simulink model "Bdy"  (R2020b)
settings: configuration reference "unit_config" (kept outside this file)
undefined symbols (not defined in the file): Bdy_facTireFric_C, Bdy_lenRadiusWheel_C, Bdy_mEquivalentJ_C, Bdy_mVeh_C, Bdy_vsqr2frc_C
settings Model: DataDictionary=Hybrid_vehicle.sldd  SimulationMode=accelerator  Creator=Georg  LastModifiedBy=jy
settings ConfigSetRef: SourceName=unit_config

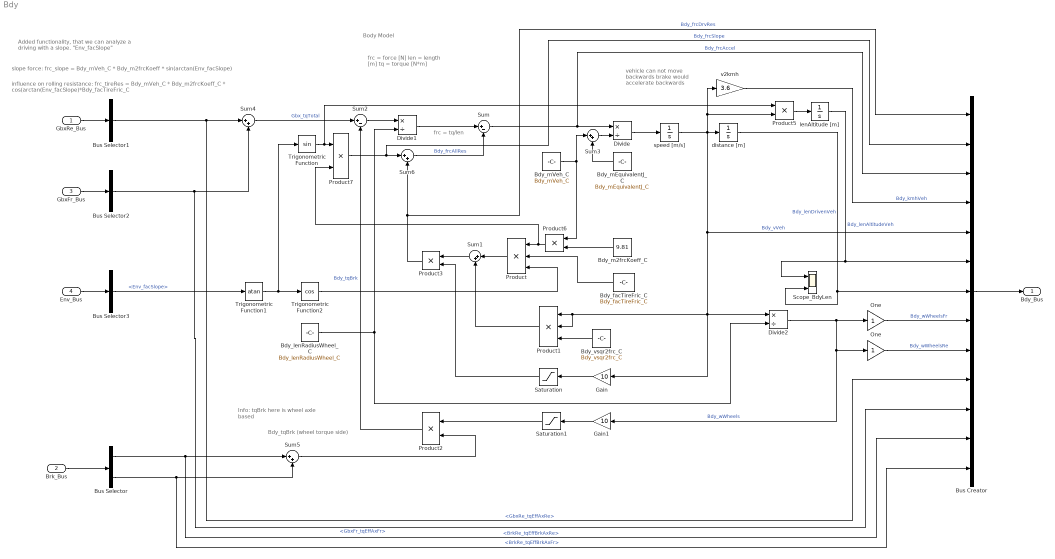
== system Bdy ==
  note: influence on rolling resistance: frc_tireRes = Bdy_mVeh_C * Bdy_m2frcKoeff_C * cos(arctan(Env_facSlope)*Bdy_facTireFric_C
  note: slope force: frc_slope = Bdy_mVeh_C * Bdy_m2frcKoeff * sin(arctan(Env_facSlope)
  note: Added functionality, that we can analyze a
      | driving with a slope.  "Env_facSlope"
  note: Info:
      | tqBrk here is wheel axle based
  note: Body Model
  note: Bdy_tqBrk
      | (wheel torque side)
  note: frc = tq/len
  note: vehicle can not
      | move backwards
      | brake would accelerate
      | backwards
  note: frc = force [N]
      | len = length [m]
      | tq = torque [N*m]
  GbxRe_Bus : Inport
  Brk_Bus : Inport  Port=2
  GbxFr_Bus : Inport  Port=3
  Env_Bus : Inport  Port=4
  Bdy_facTireFric_C : Constant  Value=Bdy_facTireFric_C
  Bdy_lenRadiusWheel_C : Constant  Value=Bdy_lenRadiusWheel_C
  Bdy_m2frcKoeff_C : Constant  Value=9.81
  Bdy_mEquivalentJ_C : Constant  Value=Bdy_mEquivalentJ_C
  Bdy_mVeh_C : Constant  Value=Bdy_mVeh_C
  Bdy_vsqr2frc_C : Constant  Value=Bdy_vsqr2frc_C
  Bus Creator : BusCreator  Inputs=13
  Bus Selector : BusSelector  OutputSignals=BrkRe_tqEffBrkAxRe,BrkRe_tqEffBrkAxFr
  Bus Selector1 : BusSelector  OutputSignals=GbxRe_tqEffAxRe
  Bus Selector2 : BusSelector  OutputSignals=GbxFr_tqEffAxFr
  Bus Selector3 : BusSelector  OutputSignals=Env_facSlope
  Divide : Product  Inputs=*/
  Divide1 : Product  Inputs=*/
  Divide2 : Product  Inputs=*/
  Gain : Gain  Gain=10
  Gain1 : Gain  Gain=10
  One : Gain
  "One " : Gain
  Product : Product  Inputs=3  RndMeth=Zero
  Product1 : Product  Inputs=3  RndMeth=Zero
  Product2 : Product  RndMeth=Zero
  Product3 : Product  RndMeth=Zero
  Product5 : Product
  Product6 : Product  RndMeth=Zero
  Product7 : Product
  Saturation : Saturate  UpperLimit=1  LowerLimit=-1
  Saturation1 : Saturate  UpperLimit=1  LowerLimit=-1
  "Scope_BdyLen  " : Scope  NumInputPorts=2
  Sum : Sum  Inputs=|+-
  Sum{1,3..6} (5 alike) : Sum  Inputs=|++
  Sum2 : Sum  Inputs=|+-
  Trigonometric Function : Trigonometry
  Trigonometric Function1 : Trigonometry  Operator=atan
  Trigonometric Function2 : Trigonometry  Operator=cos
  distance [m] : Integrator
  lenAltitude [m] : Integrator
  speed [m/s] : Integrator  LimitOutput=on  LowerSaturationLimit=0
  v2kmh : Gain  Gain=3.6
  Bdy_Bus : Outport  VectorParamsAs1DForOutWhenUnconnected=off
  wires:
  Divide/1 -> speed [m/s]/1
  Product6/1 -> Product7/2, Product/1
  lenAltitude [m]/1 -> "Scope_BdyLen  "/1, Bus Creator/6  "Bdy_lenAltitudeVeh"
  Product5/1 -> lenAltitude [m]/1
  Trigonometric Function2/1 -> Product/3
  One/1 -> Bus Creator/9  "Bdy_wWheelsRe"
  Bdy_lenRadiusWheel_C/1 -> Divide2/2, Divide1/2
  GbxFr_Bus/1 -> Bus Selector2/1
  Sum6/1 -> Sum/2  "Bdy_frcAllRes"
  Product/1 -> Sum1/1
  Trigonometric Function/1 -> Product5/1, Product7/1
  Bdy_mEquivalentJ_C/1 -> Sum3/2
  Trigonometric Function1/1 -> Trigonometric Function2/1, Trigonometric Function/1
  Saturation1/1 -> Product2/1
  Bus Selector3/1 -> Trigonometric Function1/1  "<Env_facSlope>"
  Brk_Bus/1 -> Bus Selector/1
  Bdy_facTireFric_C/1 -> Product/2
  Product1/1 -> Sum1/2
  Gain1/1 -> Saturation1/1
  Sum1/1 -> Product3/1
  "One "/1 -> Bus Creator/8  "Bdy_wWheelsFr"
  Sum2/1 -> Divide1/1
  Saturation/1 -> Product3/2
  Bdy_mVeh_C/1 -> Product6/1, Sum3/1
  Gain/1 -> Saturation/1
  Sum3/1 -> Divide/2
  Bdy_vsqr2frc_C/1 -> Product1/3
  Bdy_m2frcKoeff_C/1 -> Product6/2
  speed [m/s]/1 -> Product5/2, v2kmh/1, distance [m]/1, Product1/1, Product1/2, Gain/1, Divide2/1, Bus Creator/5  "Bdy_vVeh"
  Env_Bus/1 -> Bus Selector3/1
  Bus Selector/1 -> Bus Creator/12, Sum5/1  "<BrkRe_tqEffBrkAxRe>"
  Bus Selector/2 -> Bus Creator/13, Sum5/2  "<BrkRe_tqEffBrkAxFr>"
  Bus Creator/1 -> Bdy_Bus/1
  GbxRe_Bus/1 -> Bus Selector1/1
  Sum/1 -> Divide/1, Bus Creator/3  "Bdy_frcAccel"
  Divide2/1 -> One/1, Gain1/1, "One "/1  "Bdy_wWheels"
  Product3/1 -> Sum6/2, Bus Creator/1  "Bdy_frcDrvRes"
  Sum4/1 -> Sum2/1  "Gbx_tqTotal"
  Sum5/1 -> Product2/2
  Product2/1 -> Sum2/2  "Bdy_tqBrk"
  distance [m]/1 -> "Scope_BdyLen  "/2, Bus Creator/7  "Bdy_lenDrivenVeh"
  Product7/1 -> Bus Creator/2, Sum6/1  "Bdy_frcSlope"
  Bus Selector2/1 -> Sum4/2, Bus Creator/11  "<GbxFr_tqEffAxFr>"
  Bus Selector1/1 -> Sum4/1, Bus Creator/10  "<GbxRe_tqEffAxRe>"
  Divide1/1 -> Sum/1
  v2kmh/1 -> Bus Creator/4  "Bdy_kmhVeh"
